simulink model "RoomFloorHeating_Compare"  (Simulink 7.6)
settings: Solver=ode23t  StartTime=0.0  StopTime=24*3600  RelTol=1e-3
libraries: carnot x46
settings Model: Creator=drhf  LastModifiedBy=drhf

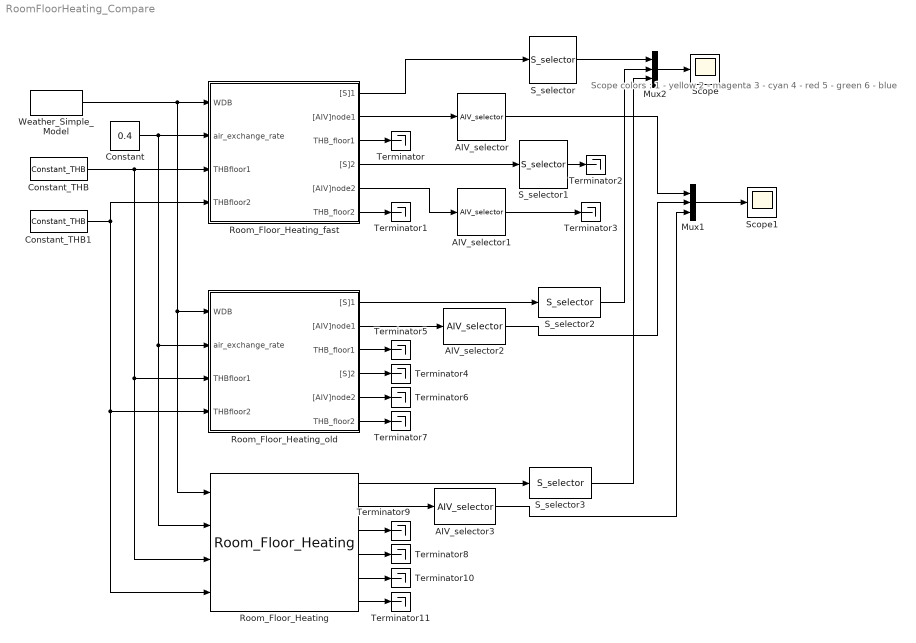
== system RoomFloorHeating_Compare ==
  note: Scope colors :
      | 1 - yellow
      | 2 - magenta
      | 3 - cyan
      | 4 - red
      | 5 - green
      | 6 - blue
  AIV_selector{,1..3} (4 alike) : carnot/Outputs/AIV_selector  SystemSampleTime=-1  e1=on  e2=on  e3=on  e4=off  e5=off  e6=off  e7=off  e8=off  e9=off
  Constant : Constant  Value=0.4
  Constant_THB : carnot/Source/Simple/Constant_THB  SystemSampleTime=-1  t=22  mdot=600/3600  p=1e5  mID=No Pressure Drop  fluid=water  mix=0  dia=0.02  hgt=0
  Constant_THB1 : carnot/Source/Simple/Constant_THB  SystemSampleTime=-1  t=40  mdot=600/3600  p=1e5  mID=No Pressure Drop  fluid=water  mix=0  dia=0.02  hgt=0
  Mux1 : Mux  Inputs=3
  Mux2 : Mux  Inputs=3
  Room_Floor_Heating : carnot/Load/Houses/Room_Floor_Heating  SystemSampleTime=-1  t0=20  temp_neighbour=20
  Room_Floor_Heating_fast : Subsystem  AncestorBlock=carnot/Load/Houses/Room_Floor_Heating  mask(room){t0=20, temp_neighbour=20}
      mask prompts: t0 "start temperature of rooms in °C"; temp_neighbour "temperature of rooms above and below in °C"
      mask help:
      | The block models of a heat transfer characteristic of two neighbour rooms.
      | Use "look under mask" to set up the models parameters (initial conditions,
      | floors and wall characteristics...)
      mask init:
      | AIV_neighbour = [0 temp_neighbour temp_neighbour 0 0 0 0 0 0];
      | zonefloordist2grnd = 0;
      mask Help: eval('man(''room_floor_heating'')')
      mask Display: plot(0,0,100,100,[30,30,60,60,30],[20,50,50,20,20],[47,47,56,56,47],[40,30,30,40,40],[42,42,34,34],[20,40,40,20],[62,45,28],[48,70,48])
  Room_Floor_Heating_old : Subsystem  AncestorBlock=carnot/Load/Houses/Room_Floor_Heating  mask(room){t0=20, temp_neighbour=20}
      mask prompts: t0 "start temperature of rooms in °C"; temp_neighbour "temperature of rooms above and below in °C"
      mask help:
      | The block models of a heat transfer characteristic of two neighbour rooms.
      | Use "look under mask" to set up the models parameters (initial conditions,
      | floors and wall characteristics...)
      mask init:
      | AIV_neighbour = [0 temp_neighbour temp_neighbour 0 0 0 0 0 0];
      | zonefloordist2grnd = 0;
      mask Help: eval('man(''room_floor_heating'')')
      mask Display: plot(0,0,100,100,[30,30,60,60,30],[20,50,50,20,20],[47,47,56,56,47],[40,30,30,40,40],[42,42,34,34],[20,40,40,20],[62,45,28],[48,70,48])
  S_selector{,1..3} (4 alike) : carnot/Outputs/S_selector  SystemSampleTime=-1  e1=off  e2=off  e3=off  e4=off  e5=off  e6=off  e7=on  e8=on  e9=off  e10=off  e11=off  e12=off  e13=off
  Scope : Scope
      settings: YMin=0  YMax=12
  Scope1 : Scope
  Terminator{,1..11} (12 alike) : Terminator
  Weather_Simple_Model : carnot/Weather/Weather_Simple_Model  SystemSampleTime=-1  lat=60  Ibn=900  Idg=100  tamb=5  deltaTsky=-6  rh=50  precip="10e-3/24/3600           % 10 mm in 24 h"  cloud=0.125  p=1013e2  vw=1  wdir=270
  wires:
  Weather_Simple_Model/1 -> Room_Floor_Heating_fast/1(WDB), Room_Floor_Heating_old/1(WDB), Room_Floor_Heating/1
  Constant/1 -> Room_Floor_Heating_fast/2(air_exchange_rate), Room_Floor_Heating_old/2(air_exchange_rate), Room_Floor_Heating/2
  Constant_THB/1 -> Room_Floor_Heating_fast/3(THBfloor1), Room_Floor_Heating_old/3(THBfloor1), Room_Floor_Heating/3
  Constant_THB1/1 -> Room_Floor_Heating_fast/4(THBfloor2), Room_Floor_Heating_old/4(THBfloor2), Room_Floor_Heating/4
  Room_Floor_Heating_fast/1("[S]1") -> S_selector/1
  Room_Floor_Heating_fast/2("[AIV]node1") -> AIV_selector/1
  Room_Floor_Heating_fast/5("[AIV]node2") -> AIV_selector1/1
  Room_Floor_Heating_fast/4("[S]2") -> S_selector1/1
  Room_Floor_Heating_fast/3(THB_floor1) -> Terminator/1
  Room_Floor_Heating_fast/6(THB_floor2) -> Terminator1/1
  Mux1/1 -> Scope1/1
  AIV_selector/1 -> Mux1/1
  S_selector1/1 -> Terminator2/1
  S_selector/1 -> Mux2/1
  Mux2/1 -> Scope/1
  Room_Floor_Heating_old/1("[S]1") -> S_selector2/1
  S_selector2/1 -> Mux2/2
  AIV_selector1/1 -> Terminator3/1
  Room_Floor_Heating_old/4("[S]2") -> Terminator4/1
  Room_Floor_Heating_old/3(THB_floor1) -> Terminator5/1
  Room_Floor_Heating_old/5("[AIV]node2") -> Terminator6/1
  Room_Floor_Heating_old/6(THB_floor2) -> Terminator7/1
  Room_Floor_Heating_old/2("[AIV]node1") -> AIV_selector2/1
  AIV_selector2/1 -> Mux1/2
  Room_Floor_Heating/4 -> Terminator8/1
  Room_Floor_Heating/3 -> Terminator9/1
  Room_Floor_Heating/5 -> Terminator10/1
  Room_Floor_Heating/6 -> Terminator11/1
  Room_Floor_Heating/2 -> AIV_selector3/1
  Room_Floor_Heating/1 -> S_selector3/1
  S_selector3/1 -> Mux2/3
  AIV_selector3/1 -> Mux1/3

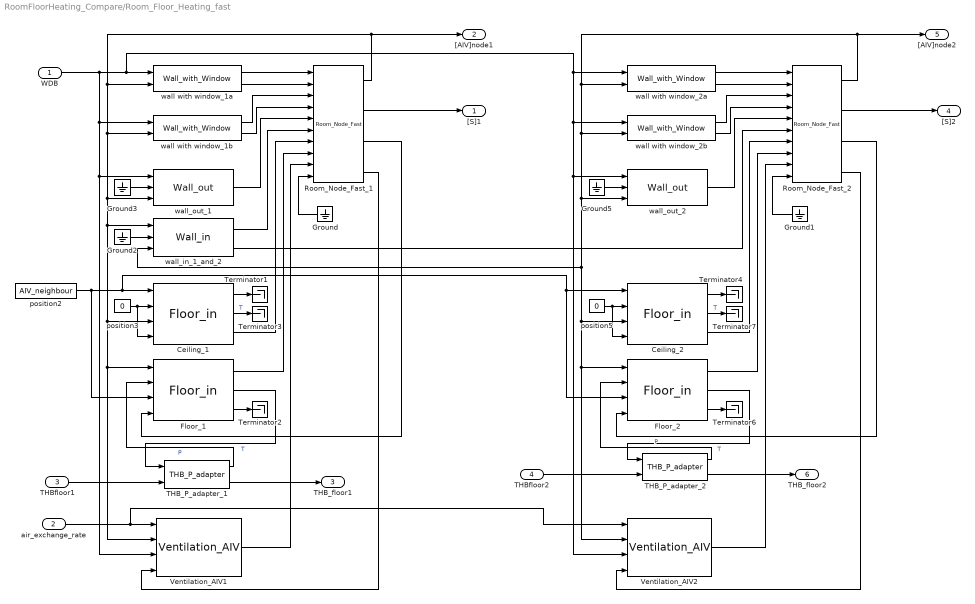
== system RoomFloorHeating_Compare/Room_Floor_Heating_fast ==
  WDB : Inport
  air_exchange_rate : Inport  Port=2
  THBfloor1 : Inport  Port=3
  THBfloor2 : Inport  Port=4
  Ceiling_1 : carnot/Load/Houses/wall_floor/Floor_in  SystemSampleTime=-1  wallsize=[5 5]  t0=20  d=[0.015 0.38 0.02]  cond=[1.4 0.79 0.7]  cwall=[0.28 0.28 0.28]*3600  rho=[2000 1800 1400]  misc=[.65 .65]  dactive=-1  tau=1000*3600
  Ceiling_2 : carnot/Load/Houses/wall_floor/Floor_in  SystemSampleTime=-1  wallsize=[5 5]  t0=20  d=[0.015 0.38 0.02]  cond=[1.4 0.79 0.7]  cwall=[0.28 0.28 0.28]*3600  rho=[2000 1800 1400]  misc=[.65 .65]  dactive=-1  tau=1000*3600
  Floor_1 : carnot/Load/Houses/wall_floor/Floor_in  SystemSampleTime=-1  wallsize=[5 5]  t0=20  d=[0.015 0.38 0.02]  cond=[1.4 0.79 0.7]  cwall=[0.28 0.28 0.28]*3600  rho=[2000 1800 1400]  misc=[.65 .65]  dactive=0.02  tau=1000*3600
  Floor_2 : carnot/Load/Houses/wall_floor/Floor_in  SystemSampleTime=-1  wallsize=[5 5]  t0=20  d=[0.015 0.38 0.02]  cond=[1.4 0.79 0.7]  cwall=[0.28 0.28 0.28]*3600  rho=[2000 1800 1400]  misc=[.65 .65]  dactive=0.02  tau=1000*3600
  Ground{,1..3,5} (5 alike) : Ground
  Room_Node_Fast_1 : carnot/Load/Houses/room_node/Room_Node_Fast  SystemSampleTime=-1  zoneairvolume=5*5*2.5  zoneheight=2.5  zonestartTEMP=20  zonestartWATER=55  timeconst=100  heatperfect=natural  lookuptime=[0 7 7 20 20 24]*3600  lookupvalue=[18 18 20 20 18 18]
  Room_Node_Fast_2 : carnot/Load/Houses/room_node/Room_Node_Fast  SystemSampleTime=-1  zoneairvolume=5*5*2.5  zoneheight=2.5  zonestartTEMP=20  zonestartWATER=55  timeconst=100  heatperfect=natural  lookuptime=[0 7 7 20 20 24]*3600  lookupvalue=[18 18 20 20 18 18]
  THB_P_adapter_1 : carnot/Load/Houses/ventilation_heating/THB_P_adapter  SystemSampleTime=-1  mass=1  ua=800*5*5/0.2*0.022*3.1415  t0=20
  THB_P_adapter_2 : carnot/Load/Houses/ventilation_heating/THB_P_adapter  SystemSampleTime=-1  mass=1  ua=800*5*5/0.2*0.022*3.1415  t0=20
  Terminator{1..4,6..7} (6 alike) : Terminator
  Ventilation_AIV1 : carnot/Source/Ventilation/Ventilation_AIV  SystemSampleTime=-1  co2=400
  Ventilation_AIV2 : carnot/Source/Ventilation/Ventilation_AIV  SystemSampleTime=-1  co2=400
  position2 : Constant  Value=AIV_neighbour
  position3 : Constant  Value=0
  position5 : Constant  Value=0
  wall with window_1a : carnot/Load/Houses/wall_floor/Wall_with_Window  SystemSampleTime=-1  wallsize=[2.5 5]  windowsize=[1 2]  frame=0.1  pos=90  t0=20  tau=1000*3600  g=0.7
  wall with window_1b : carnot/Load/Houses/wall_floor/Wall_with_Window  SystemSampleTime=-1  wallsize=[2.5 5]  windowsize=[1 2]  frame=0.1  pos=0  t0=20  tau=1000*3600  g=0.7
  wall with window_2a : carnot/Load/Houses/wall_floor/Wall_with_Window  SystemSampleTime=-1  wallsize=[2.5 5]  windowsize=[1 2]  frame=0.1  pos=-90  t0=20  tau=1000*3600  g=0.7
  wall with window_2b : carnot/Load/Houses/wall_floor/Wall_with_Window  SystemSampleTime=-1  wallsize=[2.5 5]  windowsize=[1 2]  frame=0.1  pos=0  t0=20  tau=1000*3600  g=0.7
  wall_in_1_and_2 : carnot/Load/Houses/wall_floor/Wall_in  SystemSampleTime=-1  wallsize=[2.5 5]  d=[0.015 0.38 0.02]  cond=[1.4 0.79 0.7]  cwall=[0.28 0.28 0.28]*3600  rho=[2000 1800 1400]  emission_in=.96  t0=20  tau=1000*3600  dactive=-1
  wall_out_1 : carnot/Load/Houses/wall_floor/Wall_out  SystemSampleTime=-1  wallsize=[2.5 5]  pos=180  t0=20  d=[0.1 0.38]  cond=[0.04 0.79]  cwall=[0.28 0.28]*3600  rho=[900 1800]  reflectground=0.2  abs_emiss=[0.65 0.97 0.96]  tau=1000*3600  dactive=-1
  wall_out_2 : carnot/Load/Houses/wall_floor/Wall_out  SystemSampleTime=-1  wallsize=[2.5 5]  pos=180  t0=20  d=[0.1 0.38]  cond=[0.04 0.79]  cwall=[0.28 0.28]*3600  rho=[900 1800]  reflectground=0.2  abs_emiss=[0.65 0.97 0.96]  tau=1000*3600  dactive=-1
  "[S]1" : Outport  InitialOutput=0
  "[AIV]node1" : Outport  Port=2  InitialOutput=0
  THB_floor1 : Outport  Port=3  InitialOutput=0
  "[S]2" : Outport  Port=4  InitialOutput=0
  "[AIV]node2" : Outport  Port=5  InitialOutput=0
  THB_floor2 : Outport  Port=6  InitialOutput=0
  wires:
  Room_Node_Fast_2/1 -> "[AIV]node2"/1, wall with window_2a/2, wall with window_2b/2, wall_in_1_and_2/3, Ceiling_2/3, Ventilation_AIV2/2, Floor_2/1, wall_out_2/3
  Room_Node_Fast_1/1 -> "[AIV]node1"/1, wall_out_1/3, Ventilation_AIV1/2, Floor_1/1, Ceiling_1/3, wall_in_1_and_2/1, wall with window_1b/2, wall with window_1a/2
  air_exchange_rate/1 -> Ventilation_AIV1/1, Ventilation_AIV2/1
  wall_in_1_and_2/2 -> Room_Node_Fast_2/6
  Ground5/1 -> wall_out_2/2
  Room_Node_Fast_2/3 -> Floor_2/4
  Room_Node_Fast_2/4 -> Ventilation_AIV2/4
  THB_P_adapter_2/2 -> THB_floor2/1
  THB_P_adapter_2/1 -> Floor_2/2  "P"
  Floor_2/2 -> THB_P_adapter_2/1  "T"
  THBfloor2/1 -> THB_P_adapter_2/2
  Ventilation_AIV2/1 -> Room_Node_Fast_2/9
  Ceiling_2/3 -> Room_Node_Fast_2/7
  Floor_2/1 -> Room_Node_Fast_2/8
  position5/1 -> Ceiling_2/2, Ceiling_2/4
  Floor_2/3 -> Terminator6/1
  Ceiling_2/2 -> Terminator7/1  "T"
  Ceiling_2/1 -> Terminator4/1
  Room_Node_Fast_2/2 -> "[S]2"/1
  Ground1/1 -> Room_Node_Fast_2/10
  wall with window_2b/2 -> Room_Node_Fast_2/4
  wall_out_2/1 -> Room_Node_Fast_2/5
  wall with window_2b/1 -> Room_Node_Fast_2/3
  wall with window_2a/2 -> Room_Node_Fast_2/2
  wall with window_2a/1 -> Room_Node_Fast_2/1
  position2/1 -> Floor_2/3, Ceiling_2/1, Ceiling_1/1, Floor_1/3
  Ground3/1 -> wall_out_1/2
  Ground2/1 -> wall_in_1_and_2/2
  Room_Node_Fast_1/3 -> Floor_1/4
  Room_Node_Fast_1/4 -> Ventilation_AIV1/4
  THB_P_adapter_1/2 -> THB_floor1/1
  THB_P_adapter_1/1 -> Floor_1/2  "P"
  Floor_1/2 -> THB_P_adapter_1/1  "T"
  THBfloor1/1 -> THB_P_adapter_1/2
  Ventilation_AIV1/1 -> Room_Node_Fast_1/9
  Ceiling_1/3 -> Room_Node_Fast_1/7
  Floor_1/1 -> Room_Node_Fast_1/8
  position3/1 -> Ceiling_1/4, Ceiling_1/2
  Floor_1/3 -> Terminator2/1
  Ceiling_1/2 -> Terminator3/1  "T"
  Ceiling_1/1 -> Terminator1/1
  Room_Node_Fast_1/2 -> "[S]1"/1
  Ground/1 -> Room_Node_Fast_1/10
  wall with window_1b/2 -> Room_Node_Fast_1/4
  wall_out_1/1 -> Room_Node_Fast_1/5
  wall with window_1b/1 -> Room_Node_Fast_1/3
  wall with window_1a/2 -> Room_Node_Fast_1/2
  wall with window_1a/1 -> Room_Node_Fast_1/1
  WDB/1 -> wall with window_2a/1, wall with window_2b/1, Ventilation_AIV2/3, wall_out_2/1, wall with window_1a/1, Ventilation_AIV1/3, wall_out_1/1, wall with window_1b/1
  wall_in_1_and_2/1 -> Room_Node_Fast_1/6

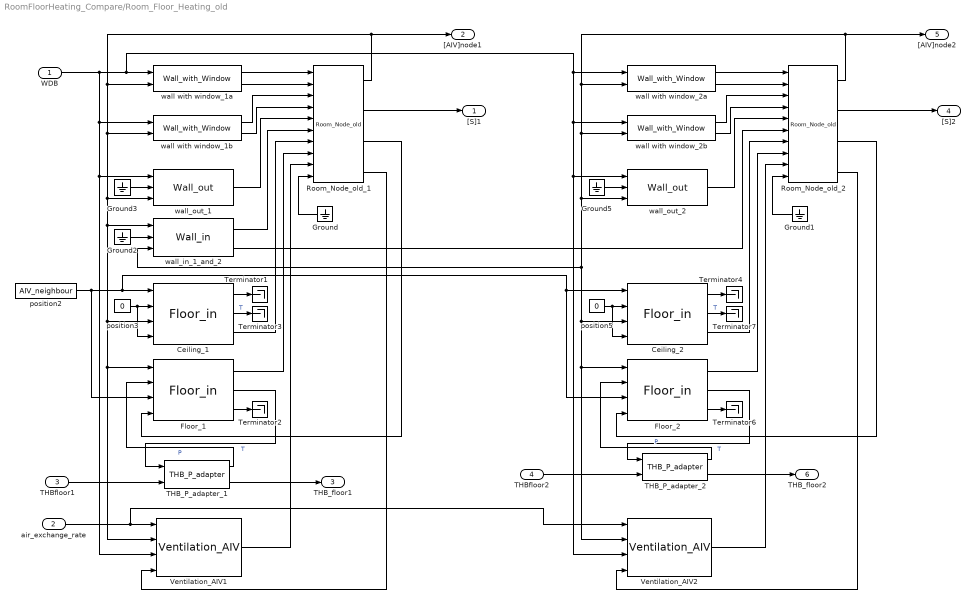
== system RoomFloorHeating_Compare/Room_Floor_Heating_old ==
  WDB : Inport
  air_exchange_rate : Inport  Port=2
  THBfloor1 : Inport  Port=3
  THBfloor2 : Inport  Port=4
  Ceiling_1 : carnot/Load/Houses/wall_floor/Floor_in  SystemSampleTime=-1  wallsize=[5 5]  t0=20  d=[0.015 0.38 0.02]  cond=[1.4 0.79 0.7]  cwall=[0.28 0.28 0.28]*3600  rho=[2000 1800 1400]  misc=[.65 .65]  dactive=-1  tau=1000*3600
  Ceiling_2 : carnot/Load/Houses/wall_floor/Floor_in  SystemSampleTime=-1  wallsize=[5 5]  t0=20  d=[0.015 0.38 0.02]  cond=[1.4 0.79 0.7]  cwall=[0.28 0.28 0.28]*3600  rho=[2000 1800 1400]  misc=[.65 .65]  dactive=-1  tau=1000*3600
  Floor_1 : carnot/Load/Houses/wall_floor/Floor_in  SystemSampleTime=-1  wallsize=[5 5]  t0=20  d=[0.015 0.38 0.02]  cond=[1.4 0.79 0.7]  cwall=[0.28 0.28 0.28]*3600  rho=[2000 1800 1400]  misc=[.65 .65]  dactive=0.02  tau=1000*3600
  Floor_2 : carnot/Load/Houses/wall_floor/Floor_in  SystemSampleTime=-1  wallsize=[5 5]  t0=20  d=[0.015 0.38 0.02]  cond=[1.4 0.79 0.7]  cwall=[0.28 0.28 0.28]*3600  rho=[2000 1800 1400]  misc=[.65 .65]  dactive=0.02  tau=1000*3600
  Ground{,1..3,5} (5 alike) : Ground
  Room_Node_old_1 : carnot/Load/Houses/room_node/Room_Node_old  SystemSampleTime=-1  zoneairvolume=5*5*2.5  zoneheight=2.5  zonestartTEMP=20  zonestartWATER=55  timeconst=100  heatperfect=natural  lookuptime=[0 7 7 20 20 24]*3600  lookupvalue=[18 18 20 20 18 18]
  Room_Node_old_2 : carnot/Load/Houses/room_node/Room_Node_old  SystemSampleTime=-1  zoneairvolume=5*5*2.5  zoneheight=2.5  zonestartTEMP=20  zonestartWATER=55  timeconst=100  heatperfect=natural  lookuptime=[0 7 7 20 20 24]*3600  lookupvalue=[18 18 20 20 18 18]
  THB_P_adapter_1 : carnot/Load/Houses/ventilation_heating/THB_P_adapter  SystemSampleTime=-1  mass=1  ua=800*5*5/0.2*0.022*3.1415  t0=20
  THB_P_adapter_2 : carnot/Load/Houses/ventilation_heating/THB_P_adapter  SystemSampleTime=-1  mass=1  ua=800*5*5/0.2*0.022*3.1415  t0=20
  Terminator{1..4,6..7} (6 alike) : Terminator
  Ventilation_AIV1 : carnot/Source/Ventilation/Ventilation_AIV  SystemSampleTime=-1  co2=400
  Ventilation_AIV2 : carnot/Source/Ventilation/Ventilation_AIV  SystemSampleTime=-1  co2=400
  position2 : Constant  Value=AIV_neighbour
  position3 : Constant  Value=0
  position5 : Constant  Value=0
  wall with window_1a : carnot/Load/Houses/wall_floor/Wall_with_Window  SystemSampleTime=-1  wallsize=[2.5 5]  windowsize=[1 2]  frame=0.1  pos=90  t0=20  tau=1000*3600  g=0.7
  wall with window_1b : carnot/Load/Houses/wall_floor/Wall_with_Window  SystemSampleTime=-1  wallsize=[2.5 5]  windowsize=[1 2]  frame=0.1  pos=0  t0=20  tau=1000*3600  g=0.7
  wall with window_2a : carnot/Load/Houses/wall_floor/Wall_with_Window  SystemSampleTime=-1  wallsize=[2.5 5]  windowsize=[1 2]  frame=0.1  pos=-90  t0=20  tau=1000*3600  g=0.7
  wall with window_2b : carnot/Load/Houses/wall_floor/Wall_with_Window  SystemSampleTime=-1  wallsize=[2.5 5]  windowsize=[1 2]  frame=0.1  pos=0  t0=20  tau=1000*3600  g=0.7
  wall_in_1_and_2 : carnot/Load/Houses/wall_floor/Wall_in  SystemSampleTime=-1  wallsize=[2.5 5]  d=[0.015 0.38 0.02]  cond=[1.4 0.79 0.7]  cwall=[0.28 0.28 0.28]*3600  rho=[2000 1800 1400]  emission_in=.96  t0=20  tau=1000*3600  dactive=-1
  wall_out_1 : carnot/Load/Houses/wall_floor/Wall_out  SystemSampleTime=-1  wallsize=[2.5 5]  pos=180  t0=20  d=[0.1 0.38]  cond=[0.04 0.79]  cwall=[0.28 0.28]*3600  rho=[900 1800]  reflectground=0.2  abs_emiss=[0.65 0.97 0.96]  tau=1000*3600  dactive=-1
  wall_out_2 : carnot/Load/Houses/wall_floor/Wall_out  SystemSampleTime=-1  wallsize=[2.5 5]  pos=180  t0=20  d=[0.1 0.38]  cond=[0.04 0.79]  cwall=[0.28 0.28]*3600  rho=[900 1800]  reflectground=0.2  abs_emiss=[0.65 0.97 0.96]  tau=1000*3600  dactive=-1
  "[S]1" : Outport  InitialOutput=0
  "[AIV]node1" : Outport  Port=2  InitialOutput=0
  THB_floor1 : Outport  Port=3  InitialOutput=0
  "[S]2" : Outport  Port=4  InitialOutput=0
  "[AIV]node2" : Outport  Port=5  InitialOutput=0
  THB_floor2 : Outport  Port=6  InitialOutput=0
  wires:
  Room_Node_old_2/1 -> "[AIV]node2"/1, wall with window_2a/2, wall with window_2b/2, wall_in_1_and_2/3, Ceiling_2/3, Ventilation_AIV2/2, Floor_2/1, wall_out_2/3
  Room_Node_old_1/1 -> "[AIV]node1"/1, wall_out_1/3, Ventilation_AIV1/2, Floor_1/1, Ceiling_1/3, wall_in_1_and_2/1, wall with window_1b/2, wall with window_1a/2
  air_exchange_rate/1 -> Ventilation_AIV1/1, Ventilation_AIV2/1
  wall_in_1_and_2/2 -> Room_Node_old_2/6
  Ground5/1 -> wall_out_2/2
  Room_Node_old_2/3 -> Floor_2/4
  Room_Node_old_2/4 -> Ventilation_AIV2/4
  THB_P_adapter_2/2 -> THB_floor2/1
  THB_P_adapter_2/1 -> Floor_2/2  "P"
  Floor_2/2 -> THB_P_adapter_2/1  "T"
  THBfloor2/1 -> THB_P_adapter_2/2
  Ventilation_AIV2/1 -> Room_Node_old_2/9
  Ceiling_2/3 -> Room_Node_old_2/7
  Floor_2/1 -> Room_Node_old_2/8
  position5/1 -> Ceiling_2/2, Ceiling_2/4
  Floor_2/3 -> Terminator6/1
  Ceiling_2/2 -> Terminator7/1  "T"
  Ceiling_2/1 -> Terminator4/1
  Room_Node_old_2/2 -> "[S]2"/1
  Ground1/1 -> Room_Node_old_2/10
  wall with window_2b/2 -> Room_Node_old_2/4
  wall_out_2/1 -> Room_Node_old_2/5
  wall with window_2b/1 -> Room_Node_old_2/3
  wall with window_2a/2 -> Room_Node_old_2/2
  wall with window_2a/1 -> Room_Node_old_2/1
  position2/1 -> Floor_2/3, Ceiling_2/1, Ceiling_1/1, Floor_1/3
  Ground3/1 -> wall_out_1/2
  Ground2/1 -> wall_in_1_and_2/2
  Room_Node_old_1/3 -> Floor_1/4
  Room_Node_old_1/4 -> Ventilation_AIV1/4
  THB_P_adapter_1/2 -> THB_floor1/1
  THB_P_adapter_1/1 -> Floor_1/2  "P"
  Floor_1/2 -> THB_P_adapter_1/1  "T"
  THBfloor1/1 -> THB_P_adapter_1/2
  Ventilation_AIV1/1 -> Room_Node_old_1/9
  Ceiling_1/3 -> Room_Node_old_1/7
  Floor_1/1 -> Room_Node_old_1/8
  position3/1 -> Ceiling_1/4, Ceiling_1/2
  Floor_1/3 -> Terminator2/1
  Ceiling_1/2 -> Terminator3/1  "T"
  Ceiling_1/1 -> Terminator1/1
  Room_Node_old_1/2 -> "[S]1"/1
  Ground/1 -> Room_Node_old_1/10
  wall with window_1b/2 -> Room_Node_old_1/4
  wall_out_1/1 -> Room_Node_old_1/5
  wall with window_1b/1 -> Room_Node_old_1/3
  wall with window_1a/2 -> Room_Node_old_1/2
  wall with window_1a/1 -> Room_Node_old_1/1
  WDB/1 -> wall with window_2a/1, wall with window_2b/1, Ventilation_AIV2/3, wall_out_2/1, wall with window_1a/1, Ventilation_AIV1/3, wall_out_1/1, wall with window_1b/1
  wall_in_1_and_2/1 -> Room_Node_old_1/6
